simulink model "Part1_II"  (R2023b)
settings: Solver=VariableStepAuto  StartTime=0.0  StopTime=1  RelTol=1e-3
undefined symbols (not defined in the file): null
libraries: dspfdesign x2, commchan3 x1
settings Model: Creator=henry  LastModifiedBy=henry

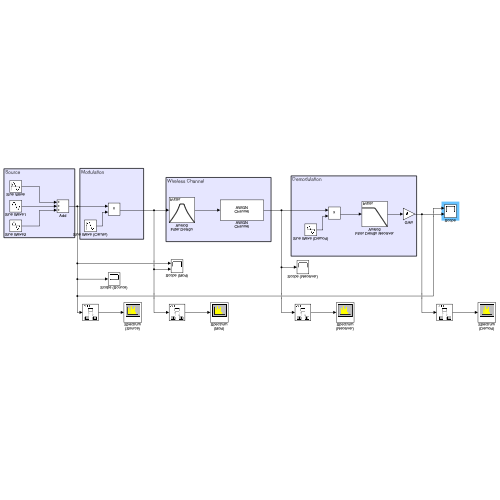
[thumbnail: Simulink's stored preview of the top-level diagram]
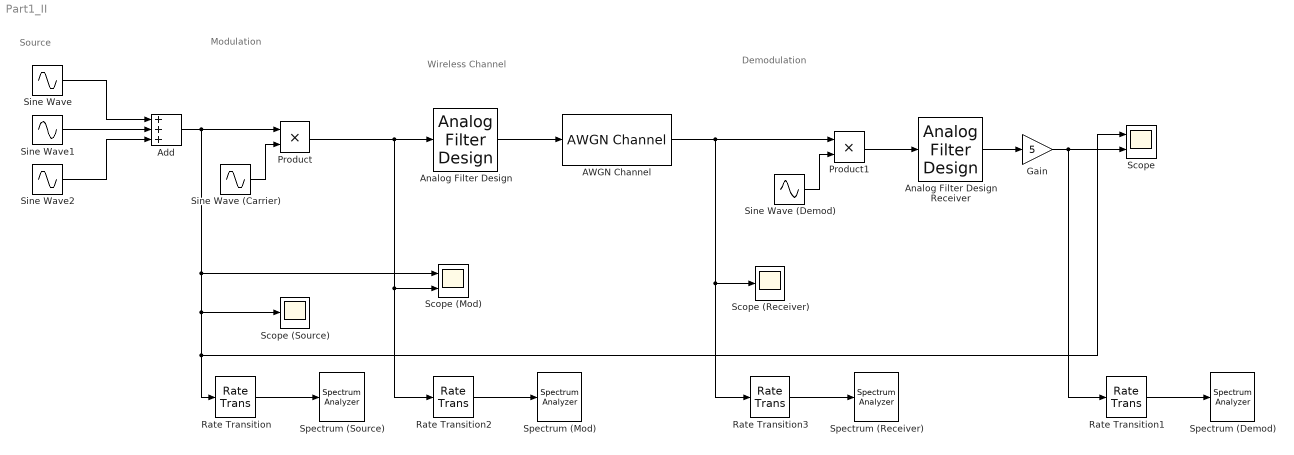
== system Part1_II ==
  note: Demodulation
  note: Modulation
  note: Wireless Channel
  note: Source
  AWGN Channel : commchan3/AWGN Channel  LegacyMode=off  NoiseMethod=Variance  noiseMode="Signal to noise ratio  (SNR)"  EbNo=10  EsNo=10  SNR=10  BitsPerSymbol=1  SignalPower=1  SamplesPerSymbol=1  SymbolPeriod=1  VarianceSource=Parameter  Variance=1e-3  RandomStream=mt19937ar with seed  Seed=100  SimulateUsing=Interpreted execution
  Add : Sum  Inputs=+++
  Analog Filter Design : dspfdesign/Analog Filter Design  method=Butterworth  filttype=Bandpass  N=8  Wlo=2e4*pi  Whi=4e4*pi  Rp=2  Rs=40
  Analog Filter Design Receiver : dspfdesign/Analog Filter Design  method=Butterworth  filttype=Lowpass  N=8  Wlo=1e4*pi  Whi=4e4*pi  Rp=2  Rs=40
  Gain : Gain  Gain=5
  Product : Product
  Product1 : Product
  Rate Transition{,1..3} (4 alike) : RateTransition  OutPortSampleTime=1/50000
  Scope : Scope  NumInputPorts=2
  Scope (Mod) : Scope  NumInputPorts=2
  Scope (Receiver) : Scope
  Scope (Source) : Scope
  Sine Wave : Sin  Amplitude=0.5  Frequency=1000*pi  SampleTime=0
  Sine Wave (Carrier) : Sin  Frequency=30000*pi  Phase=pi/2  SampleTime=0
  Sine Wave (Demod) : Sin  Frequency=30000*pi  Phase=pi/2 + pi/200  SampleTime=0
  Sine Wave1 : Sin  Amplitude=0.2  Frequency=600*pi  SampleTime=0
  Sine Wave2 : Sin  Amplitude=0.3  Frequency=1200*pi  SampleTime=0
  Spectrum (Demod) : SpectrumAnalyzer  WindowPosition=[260.000000,200.000000,800.000000,500.000000,]  Visible=on  ScopeFrameLocation=window  Span=49999.99999999999  StartFrequency=-24999.999999999996  StopFrequency=24999.999999999996  YLimits=[null,null]
  Spectrum (Mod) : SpectrumAnalyzer  WindowPosition=[320.000000,200.000000,800.000000,500.000000,]  Visible=on  ScopeFrameLocation=window  Span=49999.99999999999  StartFrequency=-24999.999999999996  StopFrequency=24999.999999999996  YLimits=[-104.42873361,24.83648092]  SelectedToolstripTab=spectrumAnalyzerToolstrip.measurementsTab
  Spectrum (Receiver) : SpectrumAnalyzer  WindowPosition=[320.000000,200.000000,800.000000,500.000000,]  Visible=on  ScopeFrameLocation=window  Span=49999.99999999999  StartFrequency=-24999.999999999996  StopFrequency=24999.999999999996  YLimits=[-39.16955483,17.62377728]
  Spectrum (Source) : SpectrumAnalyzer  WindowPosition=[320.000000,200.000000,800.000000,500.000000,]  Visible=on  ScopeFrameLocation=window  Span=49999.99999999999  StartFrequency=-24999.999999999996  StopFrequency=24999.999999999996  YLimits=[-109.32535222,32.03990898]
  wires:
  Sine Wave1/1 -> Add/2
  Sine Wave/1 -> Add/1
  Sine Wave2/1 -> Add/3
  Rate Transition/1 -> Spectrum (Source)/1
  Analog Filter Design/1 -> AWGN Channel/1
  Add/1 -> Scope/1, Rate Transition/1, Scope (Source)/1, Scope (Mod)/1, Product/1
  Sine Wave (Carrier)/1 -> Product/2
  Product/1 -> Scope (Mod)/2, Rate Transition2/1, Analog Filter Design/1
  Sine Wave (Demod)/1 -> Product1/2
  AWGN Channel/1 -> Rate Transition3/1, Scope (Receiver)/1, Product1/1
  Product1/1 -> Analog Filter Design Receiver/1
  Analog Filter Design Receiver/1 -> Gain/1
  Rate Transition2/1 -> Spectrum (Mod)/1
  Rate Transition3/1 -> Spectrum (Receiver)/1
  Rate Transition1/1 -> Spectrum (Demod)/1
  Gain/1 -> Scope/2, Rate Transition1/1
